simulink model "RAVEN_UAV_Simulation"  (R2025b)
settings: Solver=ode45  StartTime=0.0  StopTime=180  MaxStep=0.01  RelTol=1e-4
PreLoadFcn:
  | scene = uavScenario("UpdateRate", 100, "ReferenceLocation", [40.6144 -80.2007 0]);
  | plat = uavPlatform("RAVEN", scene, "ReferenceFrame", "NED");
  | updateMesh(plat, "quadrotor", {5.000}, [1 0 0], eye(4));
libraries: uavsimlib x4, uavalgslib x3, sensorbarometerlib x1
settings Model: Creator=lukewaszyn  LastModifiedBy=lukewaszyn

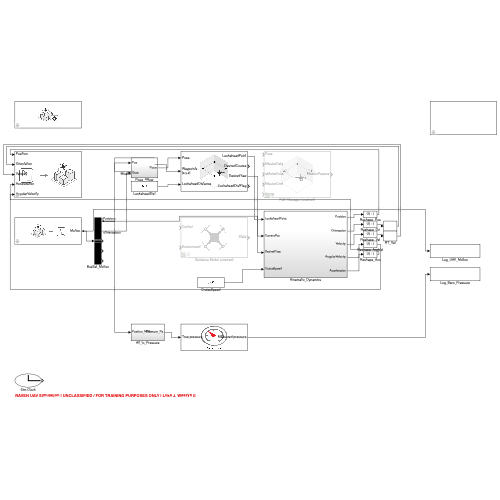
[thumbnail: Simulink's stored preview of the top-level diagram]
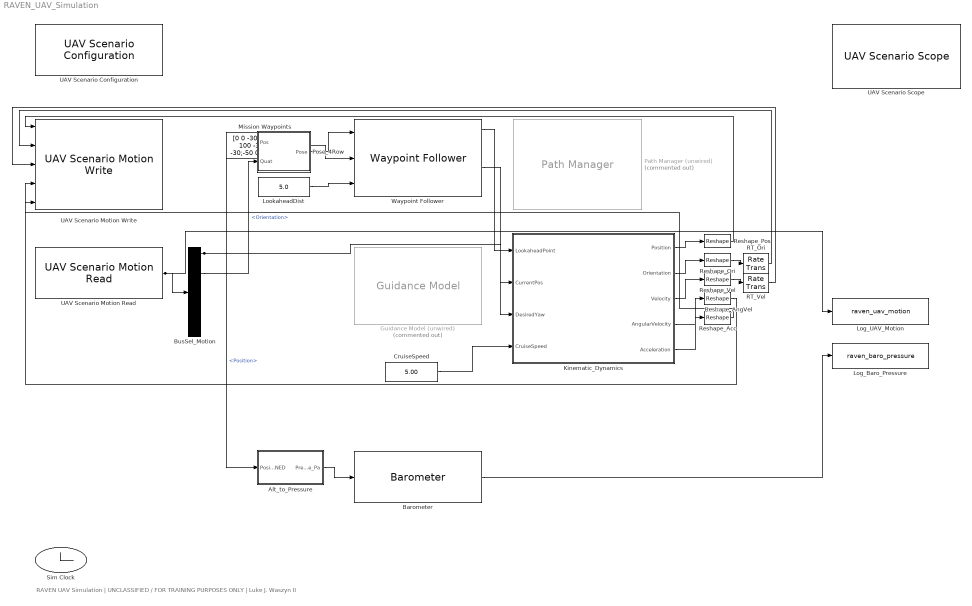
== system RAVEN_UAV_Simulation ==
  note: RAVEN UAV Simulation | UNCLASSIFIED / FOR TRAINING PURPOSES ONLY | Luke J. Waszyn II
  Alt_to_Pressure : Subsystem
  Barometer : sensorbarometerlib/Barometer  ConstantBias=0  NoiseDensity=1  BiasInstability=1  DecayFactor=0.99  SeedDouble=67  SimulateUsing=Code generation
      settings: LibrarySourceBlock=uavsimlib/Barometer
  BusSel_Motion : BusSelector  OutputSignals=Position,Orientation,Velocity,AngularVelocity,Acceleration
  CruiseSpeed : Constant  Value=5.00  OutDataTypeStr=double
  Guidance Model (unwired) : uavalgslib/Guidance Model  Commented=on  ModelType=MultirotorGuidance  NumInstances=1  SpecifiedDataType=double  SimulateUsing=Interpreted execution  InitialWorldPositionMultirotor=[0; 0; 0]  InitialWorldVelocityMultirotor=[0; 0; 0]  InitialEulerZYXMultirotor=[0; 0; 0]  InitialBodyAngularRateRPYMultirotor=[0; 0; 0]  InitialThrustMultirotor=0  InitialNorthFixedWing=0  InitialEastFixedWing=0  InitialHeightFixedWing=0  InitialAirSpeedFixedWing=0  InitialHeadingAngleFixedWing=0  InitialFlightPathAngleFixedWing=0  InitialRollAngleFixedWing=0  InitialRollAngleRateFixedWing=0  PDRollMultirotor=[3402.97,116.67]  PDPitchMultirotor=[3402.97, 116.67]  PYawRateMultirotor=1950  PThrustMultirotor=3900  MassMultirotor=1.5  PHeightFixedWing=3.9  PHeadingAngleFixedWing=3.9  PFlightPathAngleFixedWing=39  PDRollFixedWing=[3402.97, 116.67]  PAirSpeedFixedWing=1  FlightPathAngleLimitsFixedWing=[-pi/2, pi/2]  StateBusName='MultirotorGuidanceStateBus'  ControlBusName='MultirotorGuidanceControlBus'  EnvironmentBusName='MultirotorGuidanceEnvironmentBus'  DataType=double
  Kinematic_Dynamics : Subsystem
  Log_Baro_Pressure : ToWorkspace  VariableName=raven_baro_pressure  SaveFormat=Timeseries  SampleTime=-1
  Log_UAV_Motion : ToWorkspace  VariableName=raven_uav_motion  SaveFormat=Timeseries  SampleTime=-1
  LookaheadDist : Constant  Value=5.0  OutDataTypeStr=double
  Mission Waypoints : Constant  Value=[0 0 -30;50 0 -30;50 100 -30;-50 100 -30;-50 0 -30;0 0 -30]  OutDataTypeStr=double
  Path Manager (unwired) : uavalgslib/Path Manager  Commented=on  UAVType=multirotor  LoiterRadius=25  dataType=double  inputBusName='UAVPathManagerBus'  SimulateUsing=Interpreted execution
  Pose_4Row : Subsystem
  RT_Ori : RateTransition  OutPortSampleTime=0
  RT_Vel : RateTransition  OutPortSampleTime=0
  Reshape_Acc : Reshape
  Reshape_AngVel : Reshape
  Reshape_Ori : Reshape
  Reshape_Pos : Reshape
  Reshape_Vel : Reshape
  Sim Clock : Clock
  UAV Scenario Configuration : uavsimlib/UAV Scenario Configuration  Priority=-1  UAVScenarioObject=singleUAVScenario  SampleTime=0.1  UpdateParam=false  SensorMotionBusName='SensorMotionBus'  PlatformMotionBusName='PlatformMotionBus'  ScenarioMotionBusName='ScenarioMotionBus'  ScenarioMotionSignalName='ScenarioMotions'
  UAV Scenario Motion Read : uavsimlib/UAV Scenario Motion Read  Priority=1  EntityName='UAV'  ReferenceFrame=NED  OutputWind=off
  UAV Scenario Motion Write : uavsimlib/UAV Scenario Motion Write  Priority=0  PlatName='UAV'  ReferenceFrame=NED
  UAV Scenario Scope : uavsimlib/UAV Scenario Scope  Priority=1  SensorNameTable={}  SampleTime=0.1
  Waypoint Follower : uavalgslib/Waypoint Follower  UAVType=multirotor  StartFrom=first  TransitionRadiusSource=internal  TransitionRadius=10  MinLookaheadDistance=0.1  HoverAtLastWaypoint=on  YawInput=off  ShowCrossTrackErrorOutput=off  ShowStatusOutput=off  SimulateUsing=Interpreted execution
  wires:
  UAV Scenario Motion Read/1 -> BusSel_Motion/1, Log_UAV_Motion/1
  BusSel_Motion/1 -> Pose_4Row/1(Pos), Kinematic_Dynamics/2(CurrentPos), Alt_to_Pressure/1(Position_NED)  "<Position>"
  BusSel_Motion/2 -> Pose_4Row/2(Quat)  "<Orientation>"
  Pose_4Row/1(Pose) -> Waypoint Follower/1
  Mission Waypoints/1 -> Waypoint Follower/2
  LookaheadDist/1 -> Waypoint Follower/3
  Waypoint Follower/1 -> Kinematic_Dynamics/1(LookaheadPoint)
  Waypoint Follower/3 -> Kinematic_Dynamics/3(DesiredYaw)
  CruiseSpeed/1 -> Kinematic_Dynamics/4(CruiseSpeed)
  Kinematic_Dynamics/1(Position) -> Reshape_Pos/1
  Reshape_Pos/1 -> UAV Scenario Motion Write/1
  Kinematic_Dynamics/2(Orientation) -> Reshape_Ori/1
  Reshape_Ori/1 -> RT_Ori/1
  RT_Ori/1 -> UAV Scenario Motion Write/2
  Kinematic_Dynamics/3(Velocity) -> Reshape_Vel/1
  Reshape_Vel/1 -> RT_Vel/1
  RT_Vel/1 -> UAV Scenario Motion Write/3
  Kinematic_Dynamics/4(AngularVelocity) -> Reshape_AngVel/1
  Reshape_AngVel/1 -> UAV Scenario Motion Write/4
  Kinematic_Dynamics/5(Acceleration) -> Reshape_Acc/1
  Reshape_Acc/1 -> UAV Scenario Motion Write/5
  Alt_to_Pressure/1(Pressure_Pa) -> Barometer/1
  Barometer/1 -> Log_Baro_Pressure/1

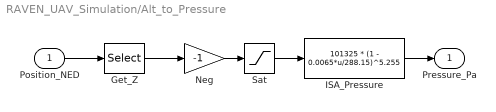
== system RAVEN_UAV_Simulation/Alt_to_Pressure ==
  Position_NED : Inport
  Get_Z : Selector  InputPortWidth=3  IndexOptions=Index vector (dialog)  Indices=3  OutputSizes=1
  ISA_Pressure : Fcn  Expr=101325 * (1 - 0.0065*u/288.15)^5.255
  Neg : Gain  Gain=-1
  Sat : Saturate  UpperLimit=inf  LowerLimit=0
  Pressure_Pa : Outport
  wires:
  Position_NED/1 -> Get_Z/1
  Get_Z/1 -> Neg/1
  Neg/1 -> Sat/1
  Sat/1 -> ISA_Pressure/1
  ISA_Pressure/1 -> Pressure_Pa/1

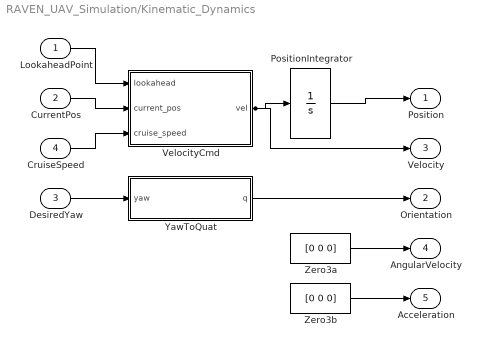
== system RAVEN_UAV_Simulation/Kinematic_Dynamics ==
  LookaheadPoint : Inport
  CurrentPos : Inport  Port=2
  DesiredYaw : Inport  Port=3
  CruiseSpeed : Inport  Port=4
  PositionIntegrator : Integrator  InitialCondition=[0;0;-30]
  VelocityCmd : MATLAB Function  TreatAsAtomicUnit=on
  YawToQuat : MATLAB Function  TreatAsAtomicUnit=on
  Zero3a : Constant  Value=[0 0 0]
  Zero3b : Constant  Value=[0 0 0]
  Position : Outport
  Orientation : Outport  Port=2
  Velocity : Outport  Port=3
  AngularVelocity : Outport  Port=4
  Acceleration : Outport  Port=5
  wires:
  LookaheadPoint/1 -> VelocityCmd/1(lookahead)
  CurrentPos/1 -> VelocityCmd/2(current_pos)
  CruiseSpeed/1 -> VelocityCmd/3(cruise_speed)
  VelocityCmd/1(vel) -> PositionIntegrator/1, Velocity/1
  PositionIntegrator/1 -> Position/1
  DesiredYaw/1 -> YawToQuat/1(yaw)
  YawToQuat/1(q) -> Orientation/1
  Zero3a/1 -> AngularVelocity/1
  Zero3b/1 -> Acceleration/1

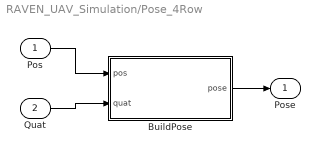
== system RAVEN_UAV_Simulation/Pose_4Row ==
  Pos : Inport
  Quat : Inport  Port=2
  BuildPose : MATLAB Function  TreatAsAtomicUnit=on
  Pose : Outport
  wires:
  Pos/1 -> BuildPose/1(pos)
  Quat/1 -> BuildPose/2(quat)
  BuildPose/1(pose) -> Pose/1

== matlab function RAVEN_UAV_Simulation/Pose_4Row/BuildPose ==
  data: pos input; pose output; quat input
function pose = build_pose(pos, quat)
p = pos(:); q = quat(:);
if any(isnan(p)) || any(isnan(q)) || norm(q) < 1e-6
    pose = [0; 0; 0; 0]; return
end
q = q / norm(q);
yaw = atan2(2*(q(1)*q(4)+q(2)*q(3)), 1-2*(q(3)^2+q(4)^2));
pose = [p(1); p(2); p(3); yaw];
end

== matlab function RAVEN_UAV_Simulation/Kinematic_Dynamics/YawToQuat ==
  data: yaw input; q output
function q = yaw_to_quat(yaw)
c = cos(yaw/2); s = sin(yaw/2);
q = [c, 0, 0, s];
end

== matlab function RAVEN_UAV_Simulation/Kinematic_Dynamics/VelocityCmd ==
  data: lookahead input; vel output; current_pos input; cruise_speed input
function vel = velocity_cmd(lookahead, current_pos, cruise_speed)
la = lookahead(:); cp = current_pos(:);
d = la - cp;
n = norm(d);
if n < 1e-6 || isnan(n)
    vel = [0; 0; 0]; return
end
vel = (d / n) * cruise_speed;
end
